simulink subsystem "k_tilde_generator"  (R2020b)
settings: Solver=VariableStepAuto  StartTime=0.0  StopTime=10.0  RelTol=1e-3
undefined symbols (not defined in the file): T_sim
settings Model: Creator=Utente CAL  LastModifiedBy=Previ

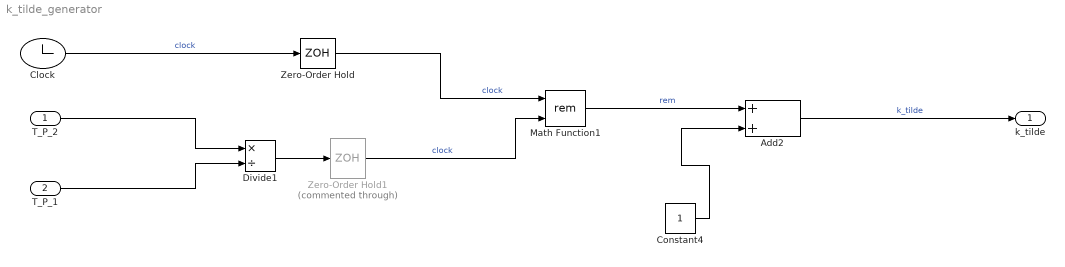
== system k_tilde_generator ==
  T_P_2 : Inport
  T_P_1 : Inport  Port=2
  Add2 : Sum  OutDataTypeStr=double
  Clock : Clock
  Constant4 : Constant  OutDataTypeStr=int32  SampleTime=-1
  Divide1 : Product  Inputs=*/
  Math Function1 : Math  Operator=rem  OutputSignalType=real  SaturateOnIntegerOverflow=on
  Zero-Order Hold : ZeroOrderHold  SampleTime=T_sim
  Zero-Order Hold1 : ZeroOrderHold  Commented=through
  k_tilde : Outport
  wires:
  Math Function1/1 -> Add2/1  "rem"
  Clock/1 -> Zero-Order Hold/1  "clock"
  Add2/1 -> k_tilde/1  "k_tilde"
  Zero-Order Hold/1 -> Math Function1/1  "clock"
  T_P_2/1 -> Divide1/1
  T_P_1/1 -> Divide1/2
  Divide1/1 -> Zero-Order Hold1/1
  Constant4/1 -> Add2/2
  Zero-Order Hold1/1 -> Math Function1/2  "clock"
